simulink model "ACC_linear"  (R2018b)
settings: Solver=ode45  StartTime=0.0  StopTime=15  RelTol=1e-6
settings Model: Creator=jinwooro  LastModifiedBy=jinwooro

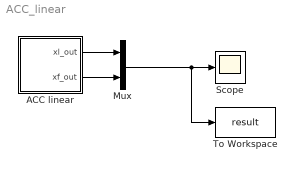
== system ACC_linear ==
  ACC linear : Stateflow chart  TreatAsAtomicUnit=on
  Mux : Mux  Inputs=2
  Scope : Scope
  To Workspace : ToWorkspace  VariableName=result  SaveFormat=Timeseries  SampleTime=-1
  wires:
  ACC linear/1(xl_out) -> Mux/1
  ACC linear/2(xf_out) -> Mux/2
  Mux/1 -> To Workspace/1, Scope/1

== stateflow chart ACC_linear/ACC linear ==
  settings: updateMethod=CONTINUOUS
  state Driving
    du:
    t_dot = 1;
    xl_dot = 7 * sin(0.5 * t) + 7;
    xf_dot = (xl - xf);
    xl_out = xl;
    xf_out = xf;
  state Collision
    du:
    t_dot = 1;
    xl_dot = 0;
    xf_dot = 0;
    xf_out = xf;
    xl_out = xl;
  (default) -> Driving : {
      | xl = 15;
      | xf = 0;
      | t = 0;
      | }
  Driving -> Collision : [(xl - xf - 5) <= 0]
  data: xf local; xl_out output; t local; xl local; xf_out output
  data xf settings: updateMethod=SF_CONTINUOUS_TIME_DATA
  data t settings: updateMethod=SF_CONTINUOUS_TIME_DATA
  data xl settings: updateMethod=SF_CONTINUOUS_TIME_DATA
